simulink model "PID_Controller"  (R2020a)
settings: Solver=VariableStepAuto  StartTime=0.0  StopTime=2  RelTol=1e-3
values from neighbouring files (symbols this model uses):
  Kd = 0.16    [DD24.sldd]
  Ki = 574.0    [DD24.sldd]
  Kp = 19.0    [DD24.sldd]
settings Model: DataDictionary=DD24.sldd  Creator=HP  LastModifiedBy=HP
settings DataIOCC: SaveOutput=off  SaveTime=off

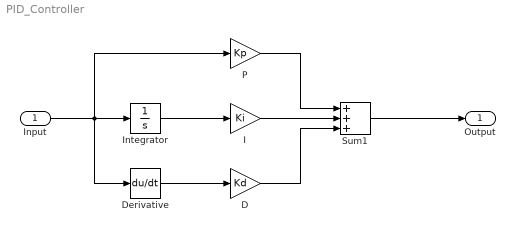
== system PID_Controller ==
  Input : Inport  OutDataTypeStr=double  PortDimensions=1  SampleTime=0
  D : Gain  Gain=Kd
  Derivative : Derivative
  I : Gain  Gain=Ki
  Integrator : Integrator
  P : Gain  Gain=Kp
  Sum1 : Sum  Inputs=+++
  Output : Outport  OutDataTypeStr=double  PortDimensions=1  SampleTime=0
  wires:
  I/1 -> Sum1/2
  Input/1 -> Derivative/1, Integrator/1, P/1
  Derivative/1 -> D/1
  P/1 -> Sum1/1
  Sum1/1 -> Output/1
  Integrator/1 -> I/1
  D/1 -> Sum1/3
